simulink model "pv_system"  (R2021a)
settings: Solver=VariableStepAuto  StartTime=0.0  StopTime=1  RelTol=1e-3
libraries: spsPVArrayLib x1, spsSeriesRLCBranchLib x1, spspowerguiLib x1
settings Model: Creator=lenovo  LastModifiedBy=ADMIN

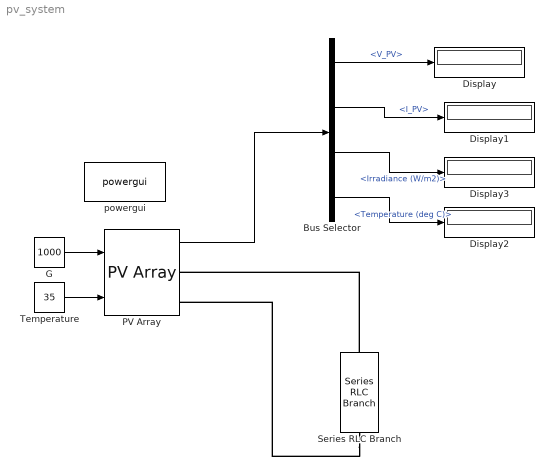
== system pv_system ==
  Bus Selector : BusSelector  OutputSignals=V_PV,I_PV,Irradiance (W/m2),Temperature (deg C)
  Display{,1..3} (4 alike) : Display
  G : Constant  Value=1000
  PV Array : spsPVArrayLib/PV Array  Npar=1  Nser=1  PlotType=array @ 1000 W/m2 & specified temperatures  S_vec="[ 1000  500  100 ]"  Temp_C_vec="[ 45 25  ]"  ModuleName=Hanwha SolarOne (Qidong) SF160-24-M150  PlotWhenSelected=off  Pm=149.988  Ncell=72  Voc=43.4  Isc=4.88  Vm=34.8  Im=4.31  beta_Voc_pc=-0.328  alpha_Isc_pc=0.033996  beta_Voc=-0.14235  alpha_Isc=0.001659  IL=4.9254  I0=4.7771e-11  nI=0.92869  Rsh=95.9331  Rs=0.79087  RobustModel=off  RobustCellTemperature=313.3991  BAL=off  Tc=1e-6  Tfilter=5e-5
  Series RLC Branch : spsSeriesRLCBranchLib/Series RLC Branch  LConnTagsString=__new0  RConnTagsString=__new0  BranchType=R  Resistance=12  Inductance=1e-3  SetiL0=off  InitialCurrent=0  Capacitance=1e-6  Setx0=off  InitialVoltage=0  Measurements=None
  Temperature : Constant  Value=35
  powergui : spspowerguiLib/powergui  Priority=1  SimulationMode=Discrete  SampleTime=1e-6  frequency=60  Iterations=50  frequencyindice=0  Pbase=100e6  ErrMax=1e-4  UnitsV=kV  UnitsW=MW  buscounter=0  FunctionMessages=off  echomessages=off  EnableUseOfTLC=off  CurrentSourceSwitches=off  DisableSnubberDevices=off  DisableRonSwitches=off  DisableVfSwitches=off  DisplayEquations=off  AutomaticDiscreteSolvers=off  SolverType=Tustin/Backward Euler (TBE)  Interpol=off  ExternalGateDelay=off  methode=off  Ts=100  x0status=blocks  SPID=on  SwTol=0  HookPort=off  NonlinearTolerance=1e-4  nMaxIteration=100  ContinueOnMaxIteration=off  RestoreLinks=warning  ResistiveCurrentMeasurement=off  Frange=[0:2:500]  Ylog=off  Xlog=on  ShowGrid=off  save=off  variable=ZData  structure=0  ZoomFFT=off  StartTime=0.0  cycles=1  DisplayStyle=1  fundamental=60  FreqAxis=off  MaxFrequency=1000  frequencyindicesteady=1  RmsSteady=1  display=off
  wires:
  PV Array/1 -> Bus Selector/1
  Bus Selector/1 -> Display/1  "<V_PV>"
  Bus Selector/2 -> Display1/1  "<I_PV>"
  Bus Selector/3 -> Display3/1  "<Irradiance (W/m2)>"
  Bus Selector/4 -> Display2/1  "<Temperature (deg C)>"
  Temperature/1 -> PV Array/2
  G/1 -> PV Array/1
  connections:
  Series RLC Branch/LConn1 -- PV Array/RConn1
  Series RLC Branch/RConn1 -- PV Array/RConn2
